simulink model "dab_modulator"  (R2026a)
settings: Solver=VariableStepAuto  StopTime=1e-3
libraries: dab_single_phase_pwm_modulator x1
settings Model: Creator=ltnbda  LastModifiedBy=ltnbda

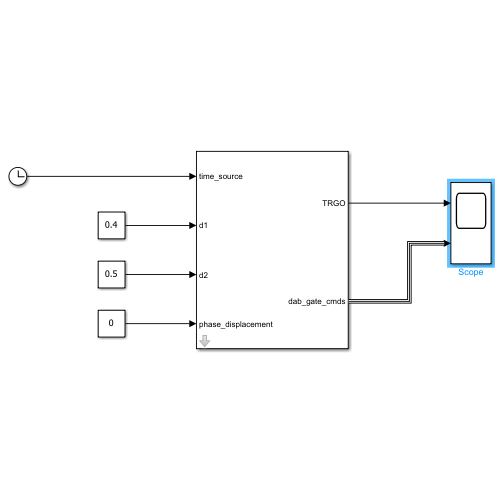
[thumbnail: Simulink's stored preview of the top-level diagram]
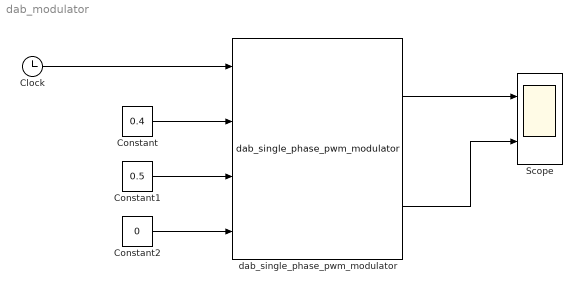
== system dab_modulator ==
  Clock : Clock
  Constant : Constant  Value=0.4
  Constant1 : Constant  Value=0.5
  Constant2 : Constant  Value=0
  Scope : Scope  NumInputPorts=2
      settings: ActiveDisplayYMinimum=-5.625  ActiveDisplayYMaximum=20.625
  dab_single_phase_pwm_modulator : dab_single_phase_pwm_modulator/dab_single_phase_pwm_modulator  fPWM_DAB=glb_time.fPWM_DAB  m_up=1  m_low=0  dead_time_DAB=glb_time.dead_time_DAB  pos_cmd_gate=18  neg_cmd_gate=-3  polarity=-1  tc=glb_time.tc  max_phase_displacement=pi/2  trgo_double_update=glb_time.TRGO_DAB_double_update
  wires:
  Constant/1 -> dab_single_phase_pwm_modulator/2
  Clock/1 -> dab_single_phase_pwm_modulator/1
  Constant1/1 -> dab_single_phase_pwm_modulator/3
  Constant2/1 -> dab_single_phase_pwm_modulator/4
  dab_single_phase_pwm_modulator/1 -> Scope/1
  dab_single_phase_pwm_modulator/2 -> Scope/2
